simulink model "PredictionRiskModule"  (R2026a)
settings: Solver=VariableStepAuto

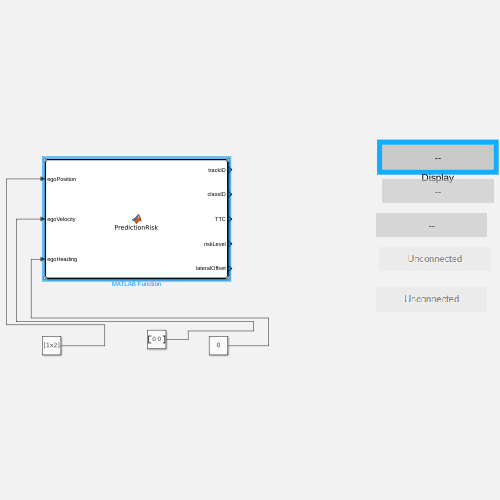
[thumbnail: Simulink's stored preview of the top-level diagram]
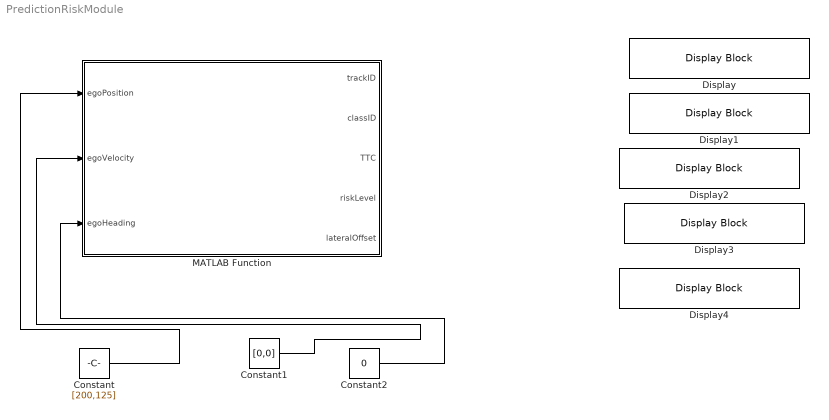
== system PredictionRiskModule ==
  Constant : Constant  Value=[200,125]
  Constant1 : Constant  Value=[0,0]
  Constant2 : Constant  Value=0
  Display{,1..4} (5 alike) : DisplayBlock  LabelPosition=Hide  Transparency=1  GridColor=[0.502, 0.502, 0.502]
  MATLAB Function : MATLAB Function  TreatAsAtomicUnit=on
  wires:
  Constant/1 -> MATLAB Function/1(egoPosition)
  Constant1/1 -> MATLAB Function/2(egoVelocity)
  Constant2/1 -> MATLAB Function/3(egoHeading)

== matlab function PredictionRiskModule/MATLAB Function ==
  data: egoPosition input; trackID output; egoVelocity input; egoHeading input; classID output; TTC output; riskLevel output; lateralOffset output
function [trackID, classID, TTC, riskLevel, lateralOffset] = ...
    PredictionRisk(egoPosition, egoVelocity, egoHeading)
%#codegen

egoState.Position = egoPosition;
egoState.Velocity = egoVelocity;
egoState.Heading = egoHeading;

detections = struct( ...
    'Frame', 1, ...
    'ClassID', 1, ...
    'Confidence', 0.95, ...
    'BoundingBox', [275 100 50 50]);

output = runPredictionRisk( ...
    detections, ...
    egoState);

decisionInput = createDecisionInput(output);

trackID = decisionInput.CriticalTrackID;
classID = decisionInput.CriticalClassID;
TTC = decisionInput.TTC;
riskLevel = decisionInput.RiskLevel;
lateralOffset = decisionInput.LateralOffset;

end
